simulink model "sm_car_4post_testrig"  (R2021b)
settings: Solver=ode23t  StartTime=0.0  StopTime=20  MaxStep=0.4  RelTol=1e-3  AbsTol=1e-3  EnableMultiTasking=on
PreLoadFcn:
  | sm_car_4post_param
  | sm_car_4post_param_posts
  | load sm_car_4post_op_01
  | load sm_car_4post_op_02
  | load sm_car_4post_op_03
  | 
  | 
  | sm_car_4post_vehicle_01_data
  | sm_car_4post_vehicle_02_data
  | sm_car_4post_vehicle_03_data
  | sm_car_4post_init_data
  | Vehicle = Vehicle_01;
  | sm_car_4post_op = sm_car_4post_op_01;
values from neighbouring files (symbols this model uses):
  brake_pressure_factor = 0.1    [sm_car_4post_param.m]
  brake_rear_factor = 0.3    [sm_car_4post_param.m]
  Init = struct    [sm_car_4post_init_data.m]
  N = 100    [sm_extr_data_cam_roller_curve.m]
  s = sin(q)    [sm_extr_data_cam_roller_curve.m]
  sm_car_4post_op_01 = simscape.op.create(simlog_sm_car_4post,20)    [sm_car_4post_gen_op.m]
  Vehicle_01 = struct    [sm_car_4post_vehicle_01_data.m]
undefined symbols (not defined in the file or in its folder): Axle, Hub, ShaftF, ShaftR, smcar_param, X, xy_data_car_side, xy_data_membrane, Y, Z
libraries: fl_lib x68, sm_lib x50, nesl_utility x40, sm_car_4post_lib x34, simulink x2
(part 4 of 4)

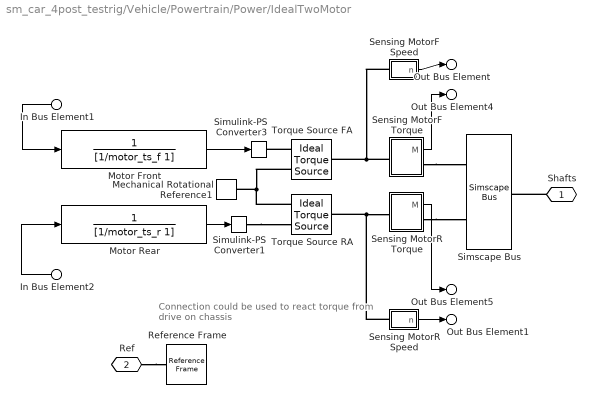
== system sm_car_4post_testrig/Vehicle/Powertrain/Power/IdealTwoMotor ==
  note: Connection could be used to
      | react torque from drive on chassis
  In Bus Element1 : Inport  PortName=CtrlBus  Element=MMotorFDemand
  In Bus Element2 : Inport  PortName=CtrlBus  Element=MMotorRDemand
  Mechanical Rotational Reference1 : fl_lib/Mechanical/Rotational Elements/Mechanical Rotational Reference
  Motor Front : TransferFcn  Denominator=[1/motor_ts_f 1]
  Motor Rear : TransferFcn  Denominator=[1/motor_ts_r 1]
  Reference Frame : sm_lib/Frames and Transforms/Reference Frame
  Sensing MotorF Speed : Subsystem
  Sensing MotorF Torque : Subsystem
  Sensing MotorR Speed : Subsystem
  Sensing MotorR Torque : Subsystem
  Simscape Bus : SimscapeBus  HierarchyStrings=ShaftF;ShaftR
  Simulink-PS Converter1 : nesl_utility/Simulink-PS Converter  PhysicalDomain=network_engine_domain  SubClassName=ps_input  LeftPortType=input  RightPortType=output  PseudoPeriodic=off  Frequencies=[]  NoiseDistribution=none  NoiseParameters=[]  Unit=1  AffineConversion=off  FilteringAndDerivatives=provide  SimscapeFilterOrder=1  InputFilterTimeConstant=0.001  UdotUserProvided=0
      settings: SourceProductBaseCode=PW,SS
  Simulink-PS Converter3 : nesl_utility/Simulink-PS Converter  PhysicalDomain=network_engine_domain  SubClassName=ps_input  LeftPortType=input  RightPortType=output  PseudoPeriodic=off  Frequencies=[]  NoiseDistribution=none  NoiseParameters=[]  Unit=1  AffineConversion=off  FilteringAndDerivatives=provide  SimscapeFilterOrder=1  InputFilterTimeConstant=0.001  UdotUserProvided=0
      settings: SourceProductBaseCode=PW,SS
  Torque Source FA : fl_lib/Mechanical/Mechanical Sources/Ideal Torque Source
  Torque Source RA : fl_lib/Mechanical/Mechanical Sources/Ideal Torque Source
  Shafts : PMIOPort  Side=Left
  Ref : PMIOPort  Port=2  Side=Right
  Out Bus Element : Outport  VectorParamsAs1DForOutWhenUnconnected=off  PortName=PowerOut  Element=nMotorF
  Out Bus Element1 : Outport  VectorParamsAs1DForOutWhenUnconnected=off  PortName=PowerOut  Element=nMotorR
  Out Bus Element4 : Outport  VectorParamsAs1DForOutWhenUnconnected=off  PortName=PowerOut  Element=MMotorF
  Out Bus Element5 : Outport  VectorParamsAs1DForOutWhenUnconnected=off  PortName=PowerOut  Element=MMotorR
  wires:
  Sensing MotorR Speed/1(n) -> Out Bus Element1/1
  Sensing MotorF Speed/1(n) -> Out Bus Element/1
  In Bus Element2/1 -> Motor Rear/1
  In Bus Element1/1 -> Motor Front/1
  Motor Front/1 -> Simulink-PS Converter3/1
  Motor Rear/1 -> Simulink-PS Converter1/1
  Sensing MotorF Torque/1(M) -> Out Bus Element4/1
  Sensing MotorR Torque/1(M) -> Out Bus Element5/1
  connections:
  Sensing MotorR Speed/LConn1 -- Torque Source RA/LConn1 -- Sensing MotorR Torque/LConn1
  Sensing MotorF Speed/LConn1 -- Sensing MotorF Torque/LConn1 -- Torque Source FA/LConn1
  Torque Source FA/RConn1 -- Simulink-PS Converter3/RConn1
  Simulink-PS Converter1/RConn1 -- Torque Source RA/RConn1
  Torque Source FA/RConn2 -- Mechanical Rotational Reference1/LConn1 -- Torque Source RA/RConn2
  Shafts/RConn1 -- Simscape Bus/RConn1
  Ref/RConn1 -- Reference Frame/RConn1
  Sensing MotorF Torque/RConn1 -- Simscape Bus/LConn1
  Sensing MotorR Torque/RConn1 -- Simscape Bus/LConn2

== system sm_car_4post_testrig/Vehicle/Powertrain/Power/IdealTwoMotor/Sensing MotorF Speed ==
  Mechanical Rotational Reference : fl_lib/Mechanical/Rotational Elements/Mechanical Rotational Reference
  Motion Sensor : fl_lib/Mechanical/Mechanical Sensors/Ideal Rotational Motion Sensor  wrap_angle=simscape.enum.onoff.off  offset=0 rad
  PS Terminator : fl_lib/Physical Signals/Sinks/PS Terminator
  PS-Simulink Converter : nesl_utility/PS-Simulink Converter  PhysicalDomain=network_engine_domain  SubClassName=ps_output  LeftPortType=input  RightPortType=output  PseudoPeriodic=off  Frequencies=[]  Unit=rad/s  AffineConversion=off
      settings: SourceProductBaseCode=PW,SS
  R : PMIOPort  Side=Left
  n : Outport  VectorParamsAs1DForOutWhenUnconnected=off
  wires:
  PS-Simulink Converter/1 -> n/1  "nMotorF"
  connections:
  Motion Sensor/RConn2 -- PS-Simulink Converter/LConn1
  Motion Sensor/RConn3 -- PS Terminator/LConn1
  Motion Sensor/LConn1 -- R/RConn1
  Motion Sensor/RConn1 -- Mechanical Rotational Reference/LConn1

== system sm_car_4post_testrig/Vehicle/Powertrain/Power/IdealTwoMotor/Sensing MotorF Torque ==
  Ideal Torque Sensor : fl_lib/Mechanical/Mechanical Sensors/Ideal Torque Sensor
  PS-Simulink Converter : nesl_utility/PS-Simulink Converter  PhysicalDomain=network_engine_domain  SubClassName=ps_output  LeftPortType=input  RightPortType=output  PseudoPeriodic=off  Frequencies=[]  Unit=N*m  AffineConversion=off
      settings: SourceProductBaseCode=PW,SS
  C : PMIOPort  Side=Right
  R : PMIOPort  Port=2  Side=Left
  M : Outport  VectorParamsAs1DForOutWhenUnconnected=off
  wires:
  PS-Simulink Converter/1 -> M/1
  connections:
  Ideal Torque Sensor/RConn2 -- PS-Simulink Converter/LConn1
  R/RConn1 -- Ideal Torque Sensor/LConn1
  Ideal Torque Sensor/RConn1 -- C/RConn1

== system sm_car_4post_testrig/Vehicle/Powertrain/Power/IdealTwoMotor/Sensing MotorR Speed ==
  Mechanical Rotational Reference : fl_lib/Mechanical/Rotational Elements/Mechanical Rotational Reference
  Motion Sensor : fl_lib/Mechanical/Mechanical Sensors/Ideal Rotational Motion Sensor  wrap_angle=simscape.enum.onoff.off  offset=0 rad
  PS Terminator : fl_lib/Physical Signals/Sinks/PS Terminator
  PS-Simulink Converter : nesl_utility/PS-Simulink Converter  PhysicalDomain=network_engine_domain  SubClassName=ps_output  LeftPortType=input  RightPortType=output  PseudoPeriodic=off  Frequencies=[]  Unit=rad/s  AffineConversion=off
      settings: SourceProductBaseCode=PW,SS
  R : PMIOPort  Side=Left
  n : Outport  VectorParamsAs1DForOutWhenUnconnected=off
  wires:
  PS-Simulink Converter/1 -> n/1  "nMotorF"
  connections:
  Motion Sensor/RConn1 -- Mechanical Rotational Reference/LConn1
  Motion Sensor/LConn1 -- R/RConn1
  Motion Sensor/RConn3 -- PS Terminator/LConn1
  Motion Sensor/RConn2 -- PS-Simulink Converter/LConn1

== system sm_car_4post_testrig/Vehicle/Powertrain/Power/IdealTwoMotor/Sensing MotorR Torque ==
  Ideal Torque Sensor : fl_lib/Mechanical/Mechanical Sensors/Ideal Torque Sensor
  PS-Simulink Converter : nesl_utility/PS-Simulink Converter  PhysicalDomain=network_engine_domain  SubClassName=ps_output  LeftPortType=input  RightPortType=output  PseudoPeriodic=off  Frequencies=[]  Unit=N*m  AffineConversion=off
      settings: SourceProductBaseCode=PW,SS
  C : PMIOPort  Side=Right
  R : PMIOPort  Port=2  Side=Left
  M : Outport  VectorParamsAs1DForOutWhenUnconnected=off
  wires:
  PS-Simulink Converter/1 -> M/1
  connections:
  Ideal Torque Sensor/RConn1 -- C/RConn1
  R/RConn1 -- Ideal Torque Sensor/LConn1
  Ideal Torque Sensor/RConn2 -- PS-Simulink Converter/LConn1
